simulink model "Quad_Nonlinear_Roll_PS"  (R2023a)
settings: Solver=ode4  StartTime=0.0  StopTime=0.5  FixedStep=0.02  RelTol=1e-3
values from neighbouring files (symbols this model uses):
  b = 1.10794e-5    (= 1.10794e-05)    [QuadParameter.m]    (also in Scenario_I.mat = 3.13e-05; Scenario_II.mat = 3.13e-05; final_PS.m = 3.6602e-06)
  d = 3.2e-6    (= 3.2e-06)    [QuadParameter.m]    (also in Scenario_I.mat; Scenario_II.mat)
  d_cg = 0.295    [QuadParameter.m]
  Gamma1 = Ixz*(Ixx - Iyy + Izz)/Gamma    [QuadConstants_v1.m]    (also in final_PS.m = 4.98954110218e-06)
  Gamma10 = (Ixx - Iyy)*Ixx + Ixz^2/Gamma    [QuadConstants_v1.m]    (also in final_PS.m = -1.44562619786e-05)
  Gamma11 = Ixx/Gamma    [QuadConstants_v1.m]    (also in final_PS.m = 24.4566929368)
  Gamma2 = Izz*(Izz - Iyy) + Ixz^2    [QuadConstants_v1.m]    (also in final_PS.m = 0.00290613207976)
  Gamma3 = Izz/Gamma    [QuadConstants_v1.m]    (also in final_PS.m = 42.1805100768)
  Gamma4 = Ixz/Gamma    [QuadConstants_v1.m]    (also in final_PS.m = 0.000237183411278)
  Gamma5 = I_rotor/Ixx    [QuadConstants_v1.m]    (also in final_PS.m = -0.0023457751623)
  Gamma6 = (Izz - Ixx)/Iyy    [QuadConstants_v1.m]    (also in final_PS.m = 2.52935414321)
  Gamma8 = 1/Iyy    [QuadConstants_v1.m]    (also in final_PS.m = 18.4688604257)
  Gamma9 = I_rotor/Iyy    [QuadConstants_v1.m]    (also in final_PS.m = 0.00216966508126)
  init_I = data(1, :)    [load_data.m]
  init_II = data(1, :)    [load_data.m]
  init_III = data(1, :)    [load_data.m]
  init_IV = data(1, :)    [load_data.m]
  init_V = data(1, :)    [load_data.m]
  Omega_I = Omega    [load_data.m]
  Omega_II = Omega    [load_data.m]
  Omega_III = Omega    [load_data.m]
  Omega_IV = Omega    [load_data.m]
  Omega_V = Omega    [load_data.m]
(part 2 of 2)

== system Quad_Nonlinear_Roll_PS/Quadcopter 3DOF Nonlinear System/Quad System/Quad System/dot(x1)/Subsystem/Subsystem1 ==
  x1 : Inport
  x2 : Inport  Port=2
  x6 : Inport  Port=3
  Cos : Trigonometry  Operator=cos
  Product1 : Product  Inputs=3
  Tan : Trigonometry  Operator=tan
  x6cos(x1)tan(x2) : Outport
  wires:
  x6/1 -> Product1/3
  x1/1 -> Cos/1
  Cos/1 -> Product1/1
  x2/1 -> Tan/1
  Product1/1 -> x6cos(x1)tan(x2)/1
  Tan/1 -> Product1/2

== system Quad_Nonlinear_Roll_PS/Quadcopter 3DOF Nonlinear System/Quad System/Quad System/dot(x2)/1/Subsystem ==
  x1 : Inport
  x5 : Inport  Port=2
  Cos : Trigonometry  Operator=cos
  Product : Product
  Out1 : Outport
  wires:
  Cos/1 -> Product/1
  Product/1 -> Out1/1
  x1/1 -> Cos/1
  x5/1 -> Product/2

== system Quad_Nonlinear_Roll_PS/Quadcopter 3DOF Nonlinear System/Quad System/Quad System/dot(x2)/Subsystem/Subsystem1 ==
  x1 : Inport
  x6 : Inport  Port=2
  Product1 : Product
  Sin : Trigonometry
  Out1 : Outport
  wires:
  x6/1 -> Product1/2
  x1/1 -> Sin/1
  Sin/1 -> Product1/1
  Product1/1 -> Out1/1

== system Quad_Nonlinear_Roll_PS/Quadcopter 3DOF Nonlinear System/Quad System/Quad System/dot(x3)/1/Subsystem ==
  x1 : Inport
  x5 : Inport  Port=2
  Product : Product
  Sin : Trigonometry
  x5sin(x1) : Outport
  wires:
  Sin/1 -> Product/1
  Product/1 -> x5sin(x1)/1
  x1/1 -> Sin/1
  x5/1 -> Product/2

== system Quad_Nonlinear_Roll_PS/Quadcopter 3DOF Nonlinear System/Quad System/Quad System/dot(x3)/Subsystem/Subsystem1 ==
  x1 : Inport
  x6 : Inport  Port=2
  Cos : Trigonometry  Operator=cos
  Product1 : Product
  Out1 : Outport
  wires:
  x6/1 -> Product1/2
  x1/1 -> Cos/1
  Cos/1 -> Product1/1
  Product1/1 -> Out1/1

== system Quad_Nonlinear_Roll_PS/Quadcopter 3DOF Nonlinear System/Quad System/Quad System/dot(x3)/Subsystem1/Sec ==
  x2 : Inport
  Constant : Constant
  Cos : Trigonometry  Operator=cos
  Divide : Product  Inputs=*/
  Sec(x2) : Outport
  wires:
  Constant/1 -> Divide/1
  Cos/1 -> Divide/2
  Divide/1 -> Sec(x2)/1
  x2/1 -> Cos/1

== system Quad_Nonlinear_Roll_PS/Quadcopter 3DOF Nonlinear System1/Quad System/Quad System/dot(x1)/1/Subsystem ==
  x1 : Inport
  x2 : Inport  Port=2
  x5 : Inport  Port=3
  Product : Product  Inputs=3
  Sin : Trigonometry
  Tan : Trigonometry  Operator=tan
  x5sin(x1)tan(x2) : Outport
  wires:
  Sin/1 -> Product/1
  x5/1 -> Product/3
  Product/1 -> x5sin(x1)tan(x2)/1
  x1/1 -> Sin/1
  x2/1 -> Tan/1
  Tan/1 -> Product/2

== system Quad_Nonlinear_Roll_PS/Quadcopter 3DOF Nonlinear System1/Quad System/Quad System/dot(x1)/Subsystem/Subsystem1 ==
  x1 : Inport
  x2 : Inport  Port=2
  x6 : Inport  Port=3
  Cos : Trigonometry  Operator=cos
  Product1 : Product  Inputs=3
  Tan : Trigonometry  Operator=tan
  x6cos(x1)tan(x2) : Outport
  wires:
  x6/1 -> Product1/3
  x1/1 -> Cos/1
  Cos/1 -> Product1/1
  x2/1 -> Tan/1
  Product1/1 -> x6cos(x1)tan(x2)/1
  Tan/1 -> Product1/2

== system Quad_Nonlinear_Roll_PS/Quadcopter 3DOF Nonlinear System1/Quad System/Quad System/dot(x2)/1/Subsystem ==
  x1 : Inport
  x5 : Inport  Port=2
  Cos : Trigonometry  Operator=cos
  Product : Product
  Out1 : Outport
  wires:
  Cos/1 -> Product/1
  Product/1 -> Out1/1
  x1/1 -> Cos/1
  x5/1 -> Product/2

== system Quad_Nonlinear_Roll_PS/Quadcopter 3DOF Nonlinear System1/Quad System/Quad System/dot(x2)/Subsystem/Subsystem1 ==
  x1 : Inport
  x6 : Inport  Port=2
  Product1 : Product
  Sin : Trigonometry
  Out1 : Outport
  wires:
  x6/1 -> Product1/2
  x1/1 -> Sin/1
  Sin/1 -> Product1/1
  Product1/1 -> Out1/1

== system Quad_Nonlinear_Roll_PS/Quadcopter 3DOF Nonlinear System1/Quad System/Quad System/dot(x3)/1/Subsystem ==
  x1 : Inport
  x5 : Inport  Port=2
  Product : Product
  Sin : Trigonometry
  x5sin(x1) : Outport
  wires:
  Sin/1 -> Product/1
  Product/1 -> x5sin(x1)/1
  x1/1 -> Sin/1
  x5/1 -> Product/2

== system Quad_Nonlinear_Roll_PS/Quadcopter 3DOF Nonlinear System1/Quad System/Quad System/dot(x3)/Subsystem/Subsystem1 ==
  x1 : Inport
  x6 : Inport  Port=2
  Cos : Trigonometry  Operator=cos
  Product1 : Product
  Out1 : Outport
  wires:
  x6/1 -> Product1/2
  x1/1 -> Cos/1
  Cos/1 -> Product1/1
  Product1/1 -> Out1/1

== system Quad_Nonlinear_Roll_PS/Quadcopter 3DOF Nonlinear System1/Quad System/Quad System/dot(x3)/Subsystem1/Sec ==
  x2 : Inport
  Constant : Constant
  Cos : Trigonometry  Operator=cos
  Divide : Product  Inputs=*/
  Sec(x2) : Outport
  wires:
  Constant/1 -> Divide/1
  Cos/1 -> Divide/2
  Divide/1 -> Sec(x2)/1
  x2/1 -> Cos/1

== system Quad_Nonlinear_Roll_PS/Quadcopter 3DOF Nonlinear System2/Quad System/Quad System/dot(x1)/1/Subsystem ==
  x1 : Inport
  x2 : Inport  Port=2
  x5 : Inport  Port=3
  Product : Product  Inputs=3
  Sin : Trigonometry
  Tan : Trigonometry  Operator=tan
  x5sin(x1)tan(x2) : Outport
  wires:
  Sin/1 -> Product/1
  x5/1 -> Product/3
  Product/1 -> x5sin(x1)tan(x2)/1
  x1/1 -> Sin/1
  x2/1 -> Tan/1
  Tan/1 -> Product/2

== system Quad_Nonlinear_Roll_PS/Quadcopter 3DOF Nonlinear System2/Quad System/Quad System/dot(x1)/Subsystem/Subsystem1 ==
  x1 : Inport
  x2 : Inport  Port=2
  x6 : Inport  Port=3
  Cos : Trigonometry  Operator=cos
  Product1 : Product  Inputs=3
  Tan : Trigonometry  Operator=tan
  x6cos(x1)tan(x2) : Outport
  wires:
  x6/1 -> Product1/3
  x1/1 -> Cos/1
  Cos/1 -> Product1/1
  x2/1 -> Tan/1
  Product1/1 -> x6cos(x1)tan(x2)/1
  Tan/1 -> Product1/2

== system Quad_Nonlinear_Roll_PS/Quadcopter 3DOF Nonlinear System2/Quad System/Quad System/dot(x2)/1/Subsystem ==
  x1 : Inport
  x5 : Inport  Port=2
  Cos : Trigonometry  Operator=cos
  Product : Product
  Out1 : Outport
  wires:
  Cos/1 -> Product/1
  Product/1 -> Out1/1
  x1/1 -> Cos/1
  x5/1 -> Product/2

== system Quad_Nonlinear_Roll_PS/Quadcopter 3DOF Nonlinear System2/Quad System/Quad System/dot(x2)/Subsystem/Subsystem1 ==
  x1 : Inport
  x6 : Inport  Port=2
  Product1 : Product
  Sin : Trigonometry
  Out1 : Outport
  wires:
  x6/1 -> Product1/2
  x1/1 -> Sin/1
  Sin/1 -> Product1/1
  Product1/1 -> Out1/1

== system Quad_Nonlinear_Roll_PS/Quadcopter 3DOF Nonlinear System2/Quad System/Quad System/dot(x3)/1/Subsystem ==
  x1 : Inport
  x5 : Inport  Port=2
  Product : Product
  Sin : Trigonometry
  x5sin(x1) : Outport
  wires:
  Sin/1 -> Product/1
  Product/1 -> x5sin(x1)/1
  x1/1 -> Sin/1
  x5/1 -> Product/2

== system Quad_Nonlinear_Roll_PS/Quadcopter 3DOF Nonlinear System2/Quad System/Quad System/dot(x3)/Subsystem/Subsystem1 ==
  x1 : Inport
  x6 : Inport  Port=2
  Cos : Trigonometry  Operator=cos
  Product1 : Product
  Out1 : Outport
  wires:
  x6/1 -> Product1/2
  x1/1 -> Cos/1
  Cos/1 -> Product1/1
  Product1/1 -> Out1/1

== system Quad_Nonlinear_Roll_PS/Quadcopter 3DOF Nonlinear System2/Quad System/Quad System/dot(x3)/Subsystem1/Sec ==
  x2 : Inport
  Constant : Constant
  Cos : Trigonometry  Operator=cos
  Divide : Product  Inputs=*/
  Sec(x2) : Outport
  wires:
  Constant/1 -> Divide/1
  Cos/1 -> Divide/2
  Divide/1 -> Sec(x2)/1
  x2/1 -> Cos/1

== system Quad_Nonlinear_Roll_PS/Quadcopter 3DOF Nonlinear System3/Quad System/Quad System/dot(x1)/1/Subsystem ==
  x1 : Inport
  x2 : Inport  Port=2
  x5 : Inport  Port=3
  Product : Product  Inputs=3
  Sin : Trigonometry
  Tan : Trigonometry  Operator=tan
  x5sin(x1)tan(x2) : Outport
  wires:
  Sin/1 -> Product/1
  x5/1 -> Product/3
  Product/1 -> x5sin(x1)tan(x2)/1
  x1/1 -> Sin/1
  x2/1 -> Tan/1
  Tan/1 -> Product/2

== system Quad_Nonlinear_Roll_PS/Quadcopter 3DOF Nonlinear System3/Quad System/Quad System/dot(x1)/Subsystem/Subsystem1 ==
  x1 : Inport
  x2 : Inport  Port=2
  x6 : Inport  Port=3
  Cos : Trigonometry  Operator=cos
  Product1 : Product  Inputs=3
  Tan : Trigonometry  Operator=tan
  x6cos(x1)tan(x2) : Outport
  wires:
  x6/1 -> Product1/3
  x1/1 -> Cos/1
  Cos/1 -> Product1/1
  x2/1 -> Tan/1
  Product1/1 -> x6cos(x1)tan(x2)/1
  Tan/1 -> Product1/2

== system Quad_Nonlinear_Roll_PS/Quadcopter 3DOF Nonlinear System3/Quad System/Quad System/dot(x2)/1/Subsystem ==
  x1 : Inport
  x5 : Inport  Port=2
  Cos : Trigonometry  Operator=cos
  Product : Product
  Out1 : Outport
  wires:
  Cos/1 -> Product/1
  Product/1 -> Out1/1
  x1/1 -> Cos/1
  x5/1 -> Product/2

== system Quad_Nonlinear_Roll_PS/Quadcopter 3DOF Nonlinear System3/Quad System/Quad System/dot(x2)/Subsystem/Subsystem1 ==
  x1 : Inport
  x6 : Inport  Port=2
  Product1 : Product
  Sin : Trigonometry
  Out1 : Outport
  wires:
  x6/1 -> Product1/2
  x1/1 -> Sin/1
  Sin/1 -> Product1/1
  Product1/1 -> Out1/1

== system Quad_Nonlinear_Roll_PS/Quadcopter 3DOF Nonlinear System3/Quad System/Quad System/dot(x3)/1/Subsystem ==
  x1 : Inport
  x5 : Inport  Port=2
  Product : Product
  Sin : Trigonometry
  x5sin(x1) : Outport
  wires:
  Sin/1 -> Product/1
  Product/1 -> x5sin(x1)/1
  x1/1 -> Sin/1
  x5/1 -> Product/2

== system Quad_Nonlinear_Roll_PS/Quadcopter 3DOF Nonlinear System3/Quad System/Quad System/dot(x3)/Subsystem/Subsystem1 ==
  x1 : Inport
  x6 : Inport  Port=2
  Cos : Trigonometry  Operator=cos
  Product1 : Product
  Out1 : Outport
  wires:
  x6/1 -> Product1/2
  x1/1 -> Cos/1
  Cos/1 -> Product1/1
  Product1/1 -> Out1/1

== system Quad_Nonlinear_Roll_PS/Quadcopter 3DOF Nonlinear System3/Quad System/Quad System/dot(x3)/Subsystem1/Sec ==
  x2 : Inport
  Constant : Constant
  Cos : Trigonometry  Operator=cos
  Divide : Product  Inputs=*/
  Sec(x2) : Outport
  wires:
  Constant/1 -> Divide/1
  Cos/1 -> Divide/2
  Divide/1 -> Sec(x2)/1
  x2/1 -> Cos/1

== system Quad_Nonlinear_Roll_PS/Quadcopter 3DOF Nonlinear System4/Quad System/Quad System/dot(x1)/1/Subsystem ==
  x1 : Inport
  x2 : Inport  Port=2
  x5 : Inport  Port=3
  Product : Product  Inputs=3
  Sin : Trigonometry
  Tan : Trigonometry  Operator=tan
  x5sin(x1)tan(x2) : Outport
  wires:
  Sin/1 -> Product/1
  x5/1 -> Product/3
  Product/1 -> x5sin(x1)tan(x2)/1
  x1/1 -> Sin/1
  x2/1 -> Tan/1
  Tan/1 -> Product/2

== system Quad_Nonlinear_Roll_PS/Quadcopter 3DOF Nonlinear System4/Quad System/Quad System/dot(x1)/Subsystem/Subsystem1 ==
  x1 : Inport
  x2 : Inport  Port=2
  x6 : Inport  Port=3
  Cos : Trigonometry  Operator=cos
  Product1 : Product  Inputs=3
  Tan : Trigonometry  Operator=tan
  x6cos(x1)tan(x2) : Outport
  wires:
  x6/1 -> Product1/3
  x1/1 -> Cos/1
  Cos/1 -> Product1/1
  x2/1 -> Tan/1
  Product1/1 -> x6cos(x1)tan(x2)/1
  Tan/1 -> Product1/2

== system Quad_Nonlinear_Roll_PS/Quadcopter 3DOF Nonlinear System4/Quad System/Quad System/dot(x2)/1/Subsystem ==
  x1 : Inport
  x5 : Inport  Port=2
  Cos : Trigonometry  Operator=cos
  Product : Product
  Out1 : Outport
  wires:
  Cos/1 -> Product/1
  Product/1 -> Out1/1
  x1/1 -> Cos/1
  x5/1 -> Product/2

== system Quad_Nonlinear_Roll_PS/Quadcopter 3DOF Nonlinear System4/Quad System/Quad System/dot(x2)/Subsystem/Subsystem1 ==
  x1 : Inport
  x6 : Inport  Port=2
  Product1 : Product
  Sin : Trigonometry
  Out1 : Outport
  wires:
  x6/1 -> Product1/2
  x1/1 -> Sin/1
  Sin/1 -> Product1/1
  Product1/1 -> Out1/1

== system Quad_Nonlinear_Roll_PS/Quadcopter 3DOF Nonlinear System4/Quad System/Quad System/dot(x3)/1/Subsystem ==
  x1 : Inport
  x5 : Inport  Port=2
  Product : Product
  Sin : Trigonometry
  x5sin(x1) : Outport
  wires:
  Sin/1 -> Product/1
  Product/1 -> x5sin(x1)/1
  x1/1 -> Sin/1
  x5/1 -> Product/2

== system Quad_Nonlinear_Roll_PS/Quadcopter 3DOF Nonlinear System4/Quad System/Quad System/dot(x3)/Subsystem/Subsystem1 ==
  x1 : Inport
  x6 : Inport  Port=2
  Cos : Trigonometry  Operator=cos
  Product1 : Product
  Out1 : Outport
  wires:
  x6/1 -> Product1/2
  x1/1 -> Cos/1
  Cos/1 -> Product1/1
  Product1/1 -> Out1/1

== system Quad_Nonlinear_Roll_PS/Quadcopter 3DOF Nonlinear System4/Quad System/Quad System/dot(x3)/Subsystem1/Sec ==
  x2 : Inport
  Constant : Constant
  Cos : Trigonometry  Operator=cos
  Divide : Product  Inputs=*/
  Sec(x2) : Outport
  wires:
  Constant/1 -> Divide/1
  Cos/1 -> Divide/2
  Divide/1 -> Sec(x2)/1
  x2/1 -> Cos/1

== matlab function Quad_Nonlinear_Roll_PS/Quadcopter 3DOF Nonlinear System4/Quad System/Quad System/MATLAB Function ==
  data: omega input; u output; b input; d input; d_cg input
function u = fcn(omega, b, d, d_cg)

u = zeros(1, 3);

u(1) = b*d_cg*(omega(2)^2 - omega(4)^2); % l
u(2) = b*d_cg*(omega(1)^2 - omega(3)^2); % m
u(3) = d*(omega(1)^2 - omega(2)^2 + omega(3)^2 - omega(4)^2); % n

== matlab function Quad_Nonlinear_Roll_PS/Quadcopter 3DOF Nonlinear System4/Quad System/Quad System/MATLAB Function1 ==
  data: X input; omega input; dot_x4 output; u input; Gamma input; dot_x5 output; dot_x6 output
function [dot_x4, dot_x5, dot_x6]  = fcn(X, omega, u, Gamma)



l = u(1);
m = u(2);
n = u(3);

p = X(4);
q = X(5);
r = X(6);

Gamma1 = Gamma(1);
Gamma2 = Gamma(2);
Gamma3 = Gamma(3);
Gamma4 = Gamma(4);
Gamma5 = Gamma(5);
Gamma6 = Gamma(6);
Gamma7 = Gamma(7);
Gamma8 = Gamma(8);
Gamma9 = Gamma(9);
Gamma10 = Gamma(10);
Gamma11 = Gamma(11);

Omega_r = -omega(1) + omega(2) - omega(3) + omega(4);

dot_x4 = Gamma1*p*q - Gamma2*q*r + Gamma3*l + Gamma4*n + Gamma5*Omega_r;
dot_x5 = Gamma6*p*r - Gamma7*(p^2-r^2) + Gamma8*m + Gamma9*Omega_r;
dot_x6 = Gamma10*p*q - Gamma1*q*r + Gamma4*l + Gamma11*n;

== matlab function Quad_Nonlinear_Roll_PS/Quadcopter 3DOF Nonlinear System1/Quad System/Quad System/MATLAB Function ==
  data: omega input; u output; b input; d input; d_cg input
function u = fcn(omega, b, d, d_cg)

u = zeros(1, 3);

u(1) = b*d_cg*(omega(2)^2 - omega(4)^2); % l
u(2) = b*d_cg*(omega(1)^2 - omega(3)^2); % m
u(3) = d*(omega(1)^2 - omega(2)^2 + omega(3)^2 - omega(4)^2); % n

== matlab function Quad_Nonlinear_Roll_PS/Quadcopter 3DOF Nonlinear System/Quad System/Quad System/MATLAB Function ==
  data: omega input; u output; b input; d input; d_cg input
function u = fcn(omega, b, d, d_cg)

u = zeros(1, 3);

u(1) = b*d_cg*(omega(2)^2 - omega(4)^2); % l
u(2) = b*d_cg*(omega(1)^2 - omega(3)^2); % m
u(3) = d*(omega(1)^2 - omega(2)^2 + omega(3)^2 - omega(4)^2); % n

== matlab function Quad_Nonlinear_Roll_PS/Quadcopter 3DOF Nonlinear System/Quad System/Quad System/MATLAB Function1 ==
  data: X input; omega input; dot_x4 output; u input; Gamma input; dot_x5 output; dot_x6 output
function [dot_x4, dot_x5, dot_x6]  = fcn(X, omega, u, Gamma)



l = u(1);
m = u(2);
n = u(3);

p = X(4);
q = X(5);
r = X(6);

Gamma1 = Gamma(1);
Gamma2 = Gamma(2);
Gamma3 = Gamma(3);
Gamma4 = Gamma(4);
Gamma5 = Gamma(5);
Gamma6 = Gamma(6);
Gamma7 = Gamma(7);
Gamma8 = Gamma(8);
Gamma9 = Gamma(9);
Gamma10 = Gamma(10);
Gamma11 = Gamma(11);

Omega_r = -omega(1) + omega(2) - omega(3) + omega(4);

dot_x4 = Gamma1*p*q - Gamma2*q*r + Gamma3*l + Gamma4*n + Gamma5*Omega_r;
dot_x5 = Gamma6*p*r - Gamma7*(p^2-r^2) + Gamma8*m + Gamma9*Omega_r;
dot_x6 = Gamma10*p*q - Gamma1*q*r + Gamma4*l + Gamma11*n;

== matlab function Quad_Nonlinear_Roll_PS/Quadcopter 3DOF Nonlinear System1/Quad System/Quad System/MATLAB Function1 ==
  data: X input; omega input; dot_x4 output; u input; Gamma input; dot_x5 output; dot_x6 output
function [dot_x4, dot_x5, dot_x6]  = fcn(X, omega, u, Gamma)



l = u(1);
m = u(2);
n = u(3);

p = X(4);
q = X(5);
r = X(6);

Gamma1 = Gamma(1);
Gamma2 = Gamma(2);
Gamma3 = Gamma(3);
Gamma4 = Gamma(4);
Gamma5 = Gamma(5);
Gamma6 = Gamma(6);
Gamma7 = Gamma(7);
Gamma8 = Gamma(8);
Gamma9 = Gamma(9);
Gamma10 = Gamma(10);
Gamma11 = Gamma(11);

Omega_r = -omega(1) + omega(2) - omega(3) + omega(4);

dot_x4 = Gamma1*p*q - Gamma2*q*r + Gamma3*l + Gamma4*n + Gamma5*Omega_r;
dot_x5 = Gamma6*p*r - Gamma7*(p^2-r^2) + Gamma8*m + Gamma9*Omega_r;
dot_x6 = Gamma10*p*q - Gamma1*q*r + Gamma4*l + Gamma11*n;

== matlab function Quad_Nonlinear_Roll_PS/Quadcopter 3DOF Nonlinear System2/Quad System/Quad System/MATLAB Function ==
  data: omega input; u output; b input; d input; d_cg input
function u = fcn(omega, b, d, d_cg)

u = zeros(1, 3);

u(1) = b*d_cg*(omega(2)^2 - omega(4)^2); % l
u(2) = b*d_cg*(omega(1)^2 - omega(3)^2); % m
u(3) = d*(omega(1)^2 - omega(2)^2 + omega(3)^2 - omega(4)^2); % n

== matlab function Quad_Nonlinear_Roll_PS/Quadcopter 3DOF Nonlinear System2/Quad System/Quad System/MATLAB Function1 ==
  data: X input; omega input; dot_x4 output; u input; Gamma input; dot_x5 output; dot_x6 output
function [dot_x4, dot_x5, dot_x6]  = fcn(X, omega, u, Gamma)



l = u(1);
m = u(2);
n = u(3);

p = X(4);
q = X(5);
r = X(6);

Gamma1 = Gamma(1);
Gamma2 = Gamma(2);
Gamma3 = Gamma(3);
Gamma4 = Gamma(4);
Gamma5 = Gamma(5);
Gamma6 = Gamma(6);
Gamma7 = Gamma(7);
Gamma8 = Gamma(8);
Gamma9 = Gamma(9);
Gamma10 = Gamma(10);
Gamma11 = Gamma(11);

Omega_r = -omega(1) + omega(2) - omega(3) + omega(4);

dot_x4 = Gamma1*p*q - Gamma2*q*r + Gamma3*l + Gamma4*n + Gamma5*Omega_r;
dot_x5 = Gamma6*p*r - Gamma7*(p^2-r^2) + Gamma8*m + Gamma9*Omega_r;
dot_x6 = Gamma10*p*q - Gamma1*q*r + Gamma4*l + Gamma11*n;

== matlab function Quad_Nonlinear_Roll_PS/Quadcopter 3DOF Nonlinear System3/Quad System/Quad System/MATLAB Function ==
  data: omega input; u output; b input; d input; d_cg input
function u = fcn(omega, b, d, d_cg)

u = zeros(1, 3);

u(1) = b*d_cg*(omega(2)^2 - omega(4)^2); % l
u(2) = b*d_cg*(omega(1)^2 - omega(3)^2); % m
u(3) = d*(omega(1)^2 - omega(2)^2 + omega(3)^2 - omega(4)^2); % n

== matlab function Quad_Nonlinear_Roll_PS/Quadcopter 3DOF Nonlinear System3/Quad System/Quad System/MATLAB Function1 ==
  data: X input; omega input; dot_x4 output; u input; Gamma input; dot_x5 output; dot_x6 output
function [dot_x4, dot_x5, dot_x6]  = fcn(X, omega, u, Gamma)



l = u(1);
m = u(2);
n = u(3);

p = X(4);
q = X(5);
r = X(6);

Gamma1 = Gamma(1);
Gamma2 = Gamma(2);
Gamma3 = Gamma(3);
Gamma4 = Gamma(4);
Gamma5 = Gamma(5);
Gamma6 = Gamma(6);
Gamma7 = Gamma(7);
Gamma8 = Gamma(8);
Gamma9 = Gamma(9);
Gamma10 = Gamma(10);
Gamma11 = Gamma(11);

Omega_r = -omega(1) + omega(2) - omega(3) + omega(4);

dot_x4 = Gamma1*p*q - Gamma2*q*r + Gamma3*l + Gamma4*n + Gamma5*Omega_r;
dot_x5 = Gamma6*p*r - Gamma7*(p^2-r^2) + Gamma8*m + Gamma9*Omega_r;
dot_x6 = Gamma10*p*q - Gamma1*q*r + Gamma4*l + Gamma11*n;
